simulink model "Harness_31_exp_rate_based"  (R2020b)
settings: Solver=FixedStepDiscrete  StartTime=0.0  StopTime=inf  FixedStep=Ts  RelTol=1e-3  EnableMultiTasking=on
PreLoadFcn:
  | Ts = 0.05;
  | Ts_1 = 0.05;   % for runnable blink_signal
  | Ts_2 = 1;       % for runnable validate_ignition
  | 
  | SetEnumTypeBlink;
undefined symbols (not defined in the file or in its folder): BlinkerValues
libraries: simulink x1
settings Model: EnablePacing=on  SimSIMDOptimization=Portable  Creator=urempel  LastModifiedBy=bnewman
settings DataIOCC: LimitDataPoints=on  SaveFormat=Array  ReturnWorkspaceOutputs=off
settings OptimizationCC: LifeSpan=1
settings DebuggingCC: SolverPrmCheckMsg=warning  AllowSymbolicDim=off  SFUnexpectedBacktrackingDiag=warning  SFNoUnconditionalDefaultTransitionDiag=warning  SFExecutionAtInitializationDiag=none  ArithmeticOperatorsInVariantConditions=warning
settings ModelReferenceCC: PropagateSignalLabelsOutOfModel=off
settings SFSimCC: SimUseLocalCustomCode=off  CustomCodeUndefinedFunction=UseInterfaceOnly
settings RTWCC: RTWUseLocalCustomCode=off
settings CodeAppCC: StateflowObjectComments=on
settings GRTTargetCC: TargetLangStandard=C89/C90 (ANSI)
settings ConfigComp: CovMetricSettings=dw  CovSaveCumulativeToWorkspaceVar=on  CovSaveSingleToWorkspaceVar=on  CovExternalEMLEnable=off  CovSFcnEnable=off

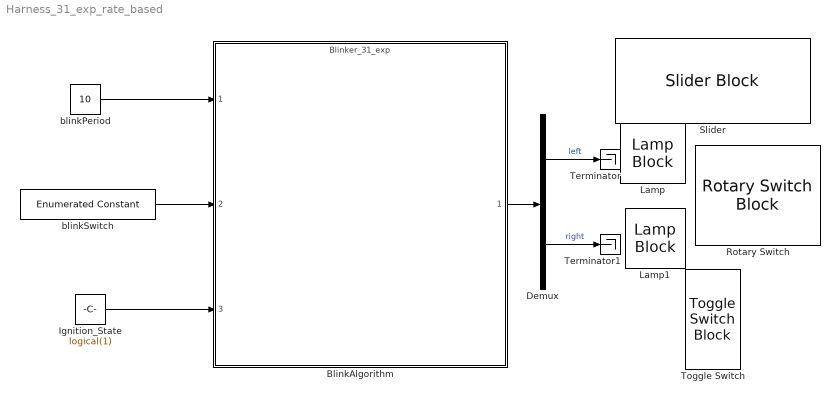
== system Harness_31_exp_rate_based ==
  BlinkAlgorithm : ModelReference  ModelNameDialog=Blinker_31_exp.slx  SimulationMode=Normal  ModelReferenceVersion=11.1
  Demux : Demux  Outputs=2
  Ignition_State : Constant  Value=logical(1)  OutDataTypeStr=boolean
      settings: AttributesFormatString=%<OutDataTypeStr>
  Lamp : LampBlock
  Lamp1 : LampBlock
  Rotary Switch : RotarySwitchBlock  UseEnumeratedDataType=on  EnumeratedDataType=BlinkerValues
      settings: Values={{'off', 'right', 'left', 'hazard'}, [0 1 2 3]}
  Slider : SliderBlock  ScaleMin=1  ScaleMax=30
  Terminator : Terminator
  Terminator1 : Terminator
  Toggle Switch : ToggleSwitchBlock
      settings: Values={{'Off', 'On'}, [0 1]}
  blinkPeriod : Constant  Value=10  OutDataTypeStr=uint32
      settings: AttributesFormatString=%<OutDataTypeStr>
  blinkSwitch : simulink/Sources/Enumerated Constant  OutDataTypeStr=Enum: BlinkerValues  Value=BlinkerValues(1)  SampleTime=inf
      settings: AttributesFormatString=%<OutDataTypeStr>
  wires:
  BlinkAlgorithm/1 -> Demux/1
  Demux/1 -> Terminator/1  "left"
  Demux/2 -> Terminator1/1  "right"
  Ignition_State/1 -> BlinkAlgorithm/3
  blinkSwitch/1 -> BlinkAlgorithm/2
  blinkPeriod/1 -> BlinkAlgorithm/1
